simulink model "demo"  (R2022a)
settings: Solver=FixedStepDiscrete  StartTime=0.0  StopTime=inf  RelTol=1e-3  EnableMultiTasking=on
InitFcn:
  | run('busObjects.m')
undefined symbols (not defined in the file or in its folder): HS, IO291
libraries: aru_toolbox x16, speedgoatlib_IO691 x10, speedgoatlib_IO291 x1
settings Model: SimulationMode=external  ExtModeEnableFloating=off  Creator=Mechatronics  LastModifiedBy=chrismailer
settings SolverCC: ConcurrentTasks=on  AlgebraicLoopSolver=TrustRegion  PositivePriorityOrder=on  InsertRTBMode=Never (minimum delay)
settings DataIOCC: SaveFormat=Array  SaveState=on  SignalLoggingName=logsOut
settings OptimizationCC: BlockReduction=off  BooleanDataType=off  OptimizeBlockIOStorage=off  BufferReuse=off  GlobalBufferReuse=off  ExpressionFolding=off  LocalBlockOutputs=off  InitFltsAndDblsToZero=on  OptimizeDataStoreBuffers=off  BusAssignmentInplaceUpdate=off
settings DebuggingCC: SaveWithParameterizedLinksMsg=none  UnderspecifiedInitializationDetection=Classic  MergeDetectMultiDrivingBlocksExec=none  CheckExecutionContextPreStartOutputMsg=on  SignalResolutionControl=TryResolveAllWithWarning  TasksWithSamePriorityMsg=none  UnconnectedInputMsg=warning  UnconnectedOutputMsg=warning  UnconnectedLineMsg=warning  SFUnexpectedBacktrackingDiag=warning  SFNoUnconditionalDefaultTransitionDiag=warning  SFExecutionAtInitializationDiag=none  SFMachineParentedDataDiag=warning  ArithmeticOperatorsInVariantConditions=warning
settings HardwareCC: ProdBitPerLong=64  ProdLongLongMode=on  ProdHWDeviceType=Intel->x86-64 (Linux 64)
settings ModelReferenceCC: PropagateSignalLabelsOutOfModel=off
settings SFSimCC: SimUseLocalCustomCode=off  SimTargetLang=C++
settings RTWCC: Description=Simulink Real-Time  SystemTargetFile=slrealtime.tlc  TemplateMakefile=slrealtime_default_tmf  RTWUseLocalCustomCode=off  Toolchain=Simulink Real-Time Toolchain  BuildConfiguration=Faster Runs  CodeExecutionProfiling=on  TargetLang=C++  DLArmComputeVersion=19.05
settings CodeAppCC: StateflowObjectComments=on
settings SimulinkRealTimeTargetCC: MATLABClassNameForMDSCustomization=Simulink.SoftwareTarget.GRTCustomization  UseGCCFastMath=on
settings ConfigComp: CovMetricSettings=dw  CovSaveCumulativeToWorkspaceVar=on  CovSaveSingleToWorkspaceVar=on  CovExternalEMLEnable=off  CovSFcnEnable=off

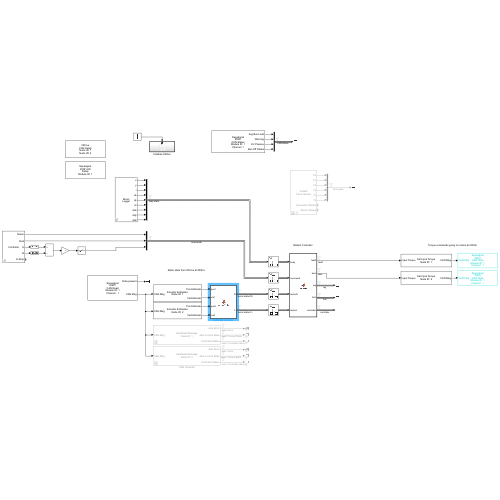
[thumbnail: Simulink's stored preview of the top-level diagram]
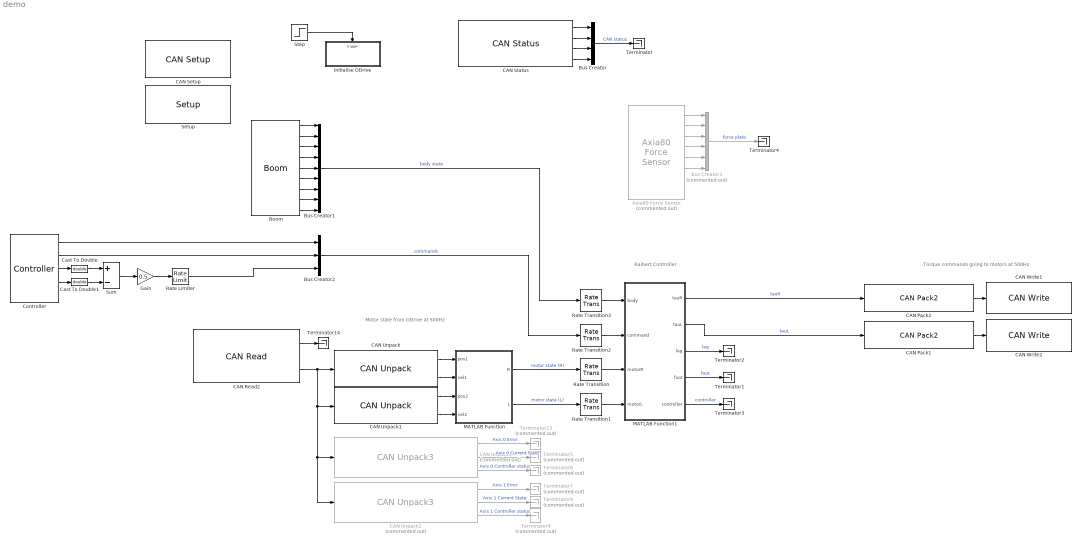
== system demo ==
  note: Torque commands going to motors at 500Hz
  note: Raibert Controller
  note: Motor state from ODrive at 500Hz
  Axia80 Force Sensor : aru_toolbox/Axia80 Force Sensor  Commented=on  resetBias=on  calibrationRangeParam=Range 0 (500N Fxy, 900N Fz, 20Nm Txyz)  sampleRateParam=975Hz  filterParam=No filtering (200Hz @ 0.5kHz, 350Hz @ 1kHz, 500Hz @ 2kHz, 1000Hz @ 4kHz)
      settings: SourceProductName=ARU Toolbox
  Boom : aru_toolbox/Boom  ts=0.001
      link override Serial Read HW FIFO: pciSlot=-1
      link override Serial Setup: pciSlot=-1
      settings: SourceProductName=ARU Toolbox
  Bus Creator : BusCreator  Inputs=4  OutDataTypeStr=Bus: CAN  NonVirtualBus=on
      settings: InheritFromInputs=off
  Bus Creator1 : BusCreator  Inputs=9  OutDataTypeStr=Bus: BodyState  NonVirtualBus=on
      settings: InheritFromInputs=off
  Bus Creator2 : BusCreator  Inputs=3  OutDataTypeStr=Bus: Command  NonVirtualBus=on
      settings: InheritFromInputs=off
  Bus Creator3 : BusCreator  Commented=on  Inputs=6  OutDataTypeStr=Bus: ForceData  NonVirtualBus=on
      settings: InheritFromInputs=off
  CAN Pack1 : aru_toolbox/ODrive/CAN Pack2  id=2
  CAN Pack2 : aru_toolbox/ODrive/CAN Pack2  id=1
  CAN Read2 : speedgoatlib_IO691/Legacy/CAN Read  id=1  ts=0.0005  channel=1  messageType=CAN  canType=CAN (HS)  BusOutput=off  initValues=[691 1 0.0005 0 1 1 0]
      settings: SourceProductName=Simulink Real-Time: Speedgoat Library
  CAN Setup : aru_toolbox/ODrive/CAN Setup  id1=1  id2=2
      settings: SourceProductName=Simulink Real-Time: Speedgoat I/O Blockset
  CAN Status : speedgoatlib_IO691/Legacy/CAN Status  moduleId=1  sampleTime=0.001  channel=1  busRecovery=Auto  arrayOutput=off  controllerCpuLoad=off  controllerLiveCount=off  initModeAct=off  avgBusLoad=on  receiving=off  RxQueueEmpty=off  dataOverrunRcv=off  rxBufferLevel=off  txPending=off  dataOverrunTx=off  txBufferLevel=off  errWarnLimit=on  errPassLimit=on  errBusOff=on  busRecoveryCounter=off  busCouplingErr=off  transceiverErr=off  opMode=off  brp=off  timeSegment1=off  timeSegment2=off  synchronisationJumpWidth=off  dataTSEG1=off  dataTSEG2=off  dataSJW=off  moduleType=691  qtyStatBlk=1  ptIdx=0  isFDMod=0
      settings: SourceProductName=Simulink Real-Time: Speedgoat I/O Blockset
  CAN Unpack : aru_toolbox/ODrive/CAN Unpack  id=1
      settings: SourceProductName=ARU Toolbox
  CAN Unpack1 : aru_toolbox/ODrive/CAN Unpack  id=2
      settings: SourceProductName=ARU Toolbox
  CAN Unpack2 : aru_toolbox/ODrive/CAN Unpack3  Commented=on  id=2
      settings: SourceProductName=ARU Toolbox
  CAN Unpack3 : aru_toolbox/ODrive/CAN Unpack3  Commented=on  id=1
      settings: SourceProductName=ARU Toolbox
  CAN Write1 : speedgoatlib_IO691/Legacy/CAN Write  id=1  ts=0.002  channel=1  messageType=CAN  BusInput=off  enableStatusPort=off  canType=CAN (HS)  initValues=[691 1 0.002 0 1 1 0 0]
      settings: SourceProductName=Simulink Real-Time: Speedgoat I/O Blockset
  CAN Write2 : speedgoatlib_IO691/Legacy/CAN Write  id=1  ts=0.002  channel=1  messageType=CAN  BusInput=off  enableStatusPort=off  canType=CAN (HS)  initValues=[691 1 0.002 0 1 1 0 0]
      settings: SourceProductName=Simulink Real-Time: Speedgoat I/O Blockset
  Cast To Double : DataTypeConversion  OutDataTypeStr=double  SaturateOnIntegerOverflow=off  RndMeth=Floor
  Cast To Double1 : DataTypeConversion  OutDataTypeStr=double  SaturateOnIntegerOverflow=off  RndMeth=Floor
  Controller : aru_toolbox/Controller
      settings: SourceProductName=ARU Toolbox
  Gain : Gain  Gain=0.5
  Initialise ODrive : Subsystem  TreatAsAtomicUnit=on
  MATLAB Function : MATLAB Function  TreatAsAtomicUnit=on
  MATLAB Function1 : MATLAB Function  TreatAsAtomicUnit=on
  Rate Limiter : RateLimiter  RisingSlewLimit=0.2  FallingSlewLimit=-0.2  SampleTimeMode=inherited
  Rate Transition{,1..3} (4 alike) : RateTransition
  "Setup " : speedgoatlib_IO291/Setup   parInternalModuleId=1  parPciSlot=-1  parModuleId=1  parModuleType=IO291-HS  parTtlDoChannels=[]  parTtlDoInitValues=1  parTtlDoReset=1  parTtlDiChannels=[1 2 3 4 5]  parIsolDiChannels=[]  parFetDoChannels=[1 2 3 4]  parFetDoInitValues=0  parFetDoReset=1
      settings: SourceProductName=Simulink Real-Time: Speedgoat I/O Blockset
  Step : Step  SampleTime=0
  Sum : Sum  Inputs=+-
  Terminator{,1..4,14} (6 alike) : Terminator
  Terminator{5..9,13} (6 alike) : Terminator  Commented=on
  wires:
  Step/1 -> Initialise ODrive/Trigger
  CAN Unpack/1 -> MATLAB Function/1(pos1)
  CAN Unpack/2 -> MATLAB Function/2(vel1)
  CAN Unpack1/1 -> MATLAB Function/3(pos2)
  CAN Unpack1/2 -> MATLAB Function/4(vel2)
  CAN Read2/2 -> CAN Unpack2/1, CAN Unpack3/1, CAN Unpack1/1, CAN Unpack/1
  CAN Status/1 -> Bus Creator/1
  CAN Status/2 -> Bus Creator/2
  CAN Status/3 -> Bus Creator/3
  CAN Status/4 -> Bus Creator/4
  CAN Unpack3/1 -> Terminator13/1  "Axis 0 Error"
  CAN Unpack3/2 -> Terminator5/1  "Axis 0 Current State"
  CAN Unpack3/3 -> Terminator6/1  "Axis 0 Controller status"
  CAN Unpack2/1 -> Terminator7/1  "Axis 1 Error"
  CAN Unpack2/2 -> Terminator8/1  "Axis 1 Current State"
  CAN Unpack2/3 -> Terminator9/1  "Axis 1 Controller status"
  CAN Read2/1 -> Terminator14/1
  MATLAB Function/1(R) -> Rate Transition/1  "motor state (R)"
  MATLAB Function/2(L) -> Rate Transition1/1  "motor state (L)"
  Bus Creator/1 -> Terminator/1  "CAN status"
  MATLAB Function1/1(tauR) -> CAN Pack2/1  "tauR"
  MATLAB Function1/2(tauL) -> CAN Pack1/1  "tauL"
  CAN Pack1/1 -> CAN Write2/1
  CAN Pack2/1 -> CAN Write1/1
  Rate Transition/1 -> MATLAB Function1/3(motorR)
  Rate Transition1/1 -> MATLAB Function1/4(motorL)
  Boom/1 -> Bus Creator1/1
  Boom/9 -> Bus Creator1/9
  Boom/2 -> Bus Creator1/2
  Boom/3 -> Bus Creator1/3
  Boom/4 -> Bus Creator1/4
  Boom/5 -> Bus Creator1/5
  Boom/6 -> Bus Creator1/6
  Boom/7 -> Bus Creator1/7
  Boom/8 -> Bus Creator1/8
  Bus Creator1/1 -> Rate Transition3/1  "body state"
  Rate Transition2/1 -> MATLAB Function1/2(command)
  Rate Transition3/1 -> MATLAB Function1/1(body)
  MATLAB Function1/4(foot) -> Terminator1/1  "foot"
  MATLAB Function1/3(leg) -> Terminator2/1  "leg"
  MATLAB Function1/5(controller) -> Terminator3/1  "controller"
  Controller/1 -> Bus Creator2/1
  Controller/2 -> Bus Creator2/2
  Bus Creator2/1 -> Rate Transition2/1  "commands"
  Axia80 Force Sensor/1 -> Bus Creator3/1
  Axia80 Force Sensor/6 -> Bus Creator3/6
  Axia80 Force Sensor/5 -> Bus Creator3/5
  Axia80 Force Sensor/4 -> Bus Creator3/4
  Axia80 Force Sensor/3 -> Bus Creator3/3
  Axia80 Force Sensor/2 -> Bus Creator3/2
  Bus Creator3/1 -> Terminator4/1  "force plate"
  Controller/3 -> Cast To Double/1
  Controller/4 -> Cast To Double1/1
  Cast To Double/1 -> Sum/1
  Cast To Double1/1 -> Sum/2
  Sum/1 -> Gain/1
  Gain/1 -> Rate Limiter/1
  Rate Limiter/1 -> Bus Creator2/3

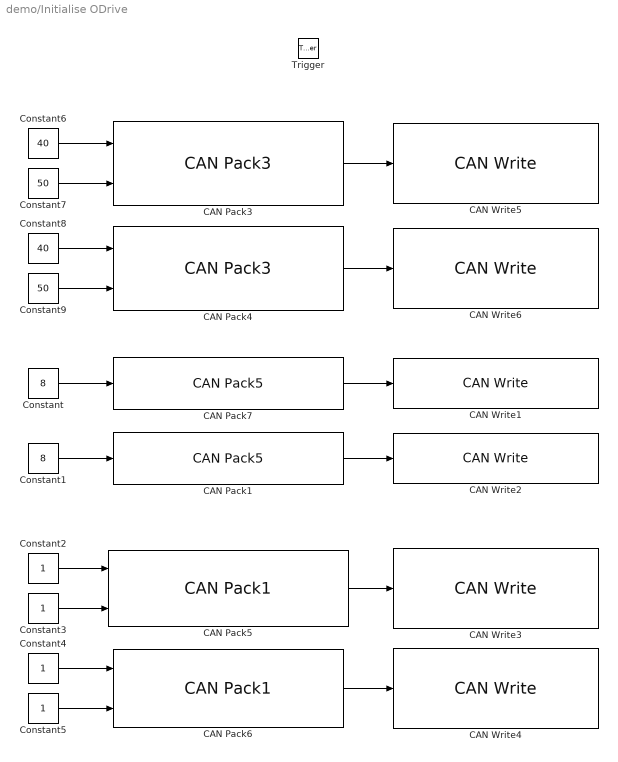
== system demo/Initialise ODrive ==
  Trigger : TriggerPort  VariantControl=Variant
  CAN Pack1 : aru_toolbox/ODrive/CAN Pack5  id=2
      settings: SourceProductName=ARU Toolbox
  CAN Pack3 : aru_toolbox/ODrive/CAN Pack3  id=1
      settings: SourceProductName=ARU Toolbox
  CAN Pack4 : aru_toolbox/ODrive/CAN Pack3  id=2
      settings: SourceProductName=ARU Toolbox
  CAN Pack5 : aru_toolbox/ODrive/CAN Pack1  id=1
      settings: SourceProductName=ARU Toolbox
  CAN Pack6 : aru_toolbox/ODrive/CAN Pack1  id=2
      settings: SourceProductName=ARU Toolbox
  CAN Pack7 : aru_toolbox/ODrive/CAN Pack5  id=1
      settings: SourceProductName=ARU Toolbox
  CAN Write{1..6} (6 alike) : speedgoatlib_IO691/Legacy/CAN Write  id=1  ts=-1  channel=1  messageType=CAN  BusInput=off  enableStatusPort=off  canType=CAN (HS)  initValues=[691 1 -1 0 1 1 0 0]
      settings: SourceProductName=Simulink Real-Time: Speedgoat I/O Blockset
  Constant : Constant  Value=8
  Constant1 : Constant  Value=8
  Constant2 : Constant  OutDataTypeStr=int32
  Constant3 : Constant
  Constant4 : Constant
  Constant5 : Constant
  Constant6 : Constant  Value=40
  Constant7 : Constant  Value=50
  Constant8 : Constant  Value=40
  Constant9 : Constant  Value=50
  wires:
  CAN Pack7/1 -> CAN Write1/1
  Constant/1 -> CAN Pack7/1
  CAN Pack1/1 -> CAN Write2/1
  Constant1/1 -> CAN Pack1/1
  Constant3/1 -> CAN Pack5/2
  Constant2/1 -> CAN Pack5/1
  Constant4/1 -> CAN Pack6/1
  Constant5/1 -> CAN Pack6/2
  CAN Pack5/1 -> CAN Write3/1
  CAN Pack6/1 -> CAN Write4/1
  Constant7/1 -> CAN Pack3/2
  Constant6/1 -> CAN Pack3/1
  Constant8/1 -> CAN Pack4/1
  Constant9/1 -> CAN Pack4/2
  CAN Pack3/1 -> CAN Write5/1
  CAN Pack4/1 -> CAN Write6/1

== matlab function demo/MATLAB Function1 ==
  data: body input Bus: BodyState; command input; motorR input Bus: MotorState; tauR output; motorL input Bus: MotorState; tauL output; leg output Bus: Leg; foot output Bus: Foot; controller output Bus: Controller
function [tauR, tauL, leg, foot, controller]   = raibert(body, command, motorR, motorL) %#codegen

leg.r = 0; leg.phi = 0; leg.dr = 0; leg.dphi = 0; leg.r0 = 0.33; leg.phi0 = -pi/2;
foot.x = 0; foot.y = 0; foot.contact = false; foot.height = 0;

[leg.r, leg.phi] = fwd_polar(motorL.q, motorR.q);
[foot.x, foot.y] = fwd_cartesian(motorL.q, motorR.q);
A = J_polar(motorL.q, motorR.q) * [motorL.w; motorR.w];
leg.dr = A(1);
leg.dphi = A(2);

% constants
N = 6; % gear ratio
dt = 0.002; % 500Hz update rate

persistent state
persistent contact_offset
persistent Ts

if isempty(state)
    state = States.Rest;
end
if isempty(contact_offset)
    contact_offset = 0;
end
if isempty(Ts)
    Ts = 0;
end

% calculate foot contact
foot.height = body.y + foot.y - contact_offset;
if (foot.height > 0.005)
    foot.contact = false;
else
    foot.contact = true;
end

% update stance duration
switch(state)
    case {States.Compression, States.Thrust, States.Unloading}
        Ts = Ts + dt;
end

% state transitions
switch(state)
    case States.Rest
        if command.start
            contact_offset = body.y + foot.y; % update foot contact offset
            state = States.Thrust;
        end
    case States.Compression
        if ((leg.dr > 0) && (leg.r < leg.r0)) % fully compressed
            contact_offset = body.y + foot.y; % update foot contact offset
            if command.stop
                state = States.Rest;
            else
                state = States.Thrust;
            end
        end
    case States.Thrust
        if (leg.r > leg.r0)
            state = States.Unloading;
        end
    case States.Unloading
        if not(foot.contact)
            Ts = min(Ts, 0.4); % record stance time
            state = States.Flight;
        end
    case States.Flight
        % foot contact check
        if (leg.dr < -1.0) && (body.dy < 0)
            contact_offset = body.y + foot.y; % update foot contact offset
            Ts = 0; % reset stance time
            state = States.Compression;
        end
end

% radial force control
switch(state)
    case States.Thrust
        F_thrust = 30;
        if command.start
            F_thrust = 60; % extra little push to get things going
        end
        Kp_r = 800; Kd_r = 0;
    case {States.Rest, States.Unloading, States.Flight}
        Kp_r = 800; Kd_r = 30; F_thrust = 0;  % damping to stop oscillation
    otherwise
        Kp_r = 800; Kd_r = 0; F_thrust = 0;
end

% phi torque control
switch(state)
    case States.Rest
        Kp_phi = 20; Kd_phi = 2;
    case States.Flight
        % adjust foot placement based on horizontal velocity
        foot_x_des = 0.25*body.dx*Ts + 0.03*(body.dx - command.dx);
        leg.phi0 = -pi/2 + asin(foot_x_des / leg.r0);
        Kp_phi = 20; Kd_phi = 1;
    otherwise
        Kp_phi = 0; Kd_phi = 0.1;
end

% polar impedance control
controller.Fr = Kp_r*(leg.r0 - leg.r) + Kd_r*(0 - leg.dr) + F_thrust;
tau = Kp_phi*(leg.phi0 - leg.phi) + Kd_phi*(0 - leg.dphi);

% ankle force to joint torques
B = transpose(J_polar(motorL.q, motorR.q)) * [controller.Fr; tau];
tauL = B(1)/N;
tauR = B(2)/N;

% update controller parameters for logging
controller.stance_time = Ts;
controller.state = state;

end

== matlab function demo/MATLAB Function ==
  data: pos1 input; R output Bus: MotorState; vel1 input; pos2 input; vel2 input; L output Bus: MotorState
function [R,L] = motor2hip(pos1, vel1, pos2, vel2) %#codegen
N = 6;
femurTaper = 0.080111; %rad

actualR = -0.2971;
actualL = -0.0555;

offsetR = femurTaper - actualR;
offsetL = pi - femurTaper - actualL;

% offsetR = 0;
% offsetL = 0;
% ODrive uses units turns and turns/s so need to explicity convert to
% radians
R.q = pos1*2*pi/N + offsetR;
R.w = vel1*2*pi/N;
L.q = pos2*2*pi/N + offsetL;
L.w = vel2*2*pi/N;
end
